simulink model "Red_problema6_Kclasica_v2"  (R2021a)
settings: Solver=ode15s  StartTime=0.0  StopTime=sim_time  RelTol=1e-3
values from neighbouring files (symbols this model uses):
  aE112 = 177.25533427288616    (= 177.255334273)    [data_run_lazo_abierto_simulink.m]    (also in inicializar_areas.m = 179.376259805; script_IMC.m = a112_f)
  aE121 = 28.272251308900536    (= 28.2722513089)    [data_run_lazo_abierto_simulink.m]    (also in inicializar_areas.m; script_IMC.m = a121_f)
  aE213 = 304.960661680865    (= 304.960661681)    [data_run_lazo_abierto_simulink.m]    (also in inicializar_areas.m; script_IMC.m = a213_f)
  aE222 = 104.78323167686085    (= 104.783231677)    [data_run_lazo_abierto_simulink.m]    (also in inicializar_areas.m = 114.075570199; script_IMC.m = a222_f)
  aEcu1 = 2.44278466343862    (= 2.44278466344)    [data_run_lazo_abierto_simulink.m]    (also in inicializar_areas.m = 4.955447053)
  aEcu2 = 9.34130944614368    (= 9.34130944614)    [data_run_lazo_abierto_simulink.m]    (also in inicializar_areas.m = 18.78773145)
  aEhu2 = 53.1053199018638    (= 53.1053199019)    [data_run_lazo_abierto_simulink.m]    (also in inicializar_areas.m = 53.1053199)
  d1_end = 0    [data_run_lazo_abierto_simulink.m]    (also in inicializar_entradas.m; pert_max.m = 0.99; script_build_tfs.m)
  d1_in = 0    [data_run_lazo_abierto_simulink.m]    (also in inicializar_entradas.m; script_build_tfs.m)
  d2_end = 0    [data_run_lazo_abierto_simulink.m]    (also in inicializar_entradas.m; pert_max.m = 0.15; script_build_tfs.m)
  d2_in = 0    [data_run_lazo_abierto_simulink.m]    (also in inicializar_entradas.m; script_build_tfs.m)
  d3_end = 0    [data_run_lazo_abierto_simulink.m]    (also in inicializar_entradas.m; pert_max.m = 0.99; script_build_tfs.m)
  d3_in = 0    [data_run_lazo_abierto_simulink.m]    (also in inicializar_entradas.m; script_build_tfs.m)
  d4_end = 0    [data_run_lazo_abierto_simulink.m]    (also in inicializar_entradas.m; pert_max.m = 0.15; script_build_tfs.m)
  d4_in = 0    [data_run_lazo_abierto_simulink.m]    (also in inicializar_entradas.m; script_build_tfs.m)
  d5_end = 0    [data_run_lazo_abierto_simulink.m]    (also in inicializar_entradas.m; pert_max.m = -0.99; script_build_tfs.m)
  d5_in = 0    [data_run_lazo_abierto_simulink.m]    (also in inicializar_entradas.m; script_build_tfs.m)
  d6_end = 0    [data_run_lazo_abierto_simulink.m]    (also in inicializar_entradas.m; pert_max.m = 0.15; script_build_tfs.m)
  d6_in = 0    [data_run_lazo_abierto_simulink.m]    (also in inicializar_entradas.m; script_build_tfs.m)
  d7_end = 0    [data_run_lazo_abierto_simulink.m]    (also in inicializar_entradas.m; pert_max.m = -0.99; script_build_tfs.m)
  d7_in = 0    [data_run_lazo_abierto_simulink.m]    (also in inicializar_entradas.m; script_build_tfs.m)
  d8_end = 0    [data_run_lazo_abierto_simulink.m]    (also in inicializar_entradas.m; pert_max.m = 0.15; script_build_tfs.m)
  d8_in = 0    [data_run_lazo_abierto_simulink.m]    (also in inicializar_entradas.m; script_build_tfs.m)
  est = 1    [data_run_lazo_abierto_simulink.m]    (also in ini_comun.m; script_build_tfs.m)
  fc1 = 20    [data_run_lazo_abierto_simulink.m]    (also in ini_comun.m; script_build_tfs.m)
  fc2 = 50    [data_run_lazo_abierto_simulink.m]    (also in ini_comun.m; script_build_tfs.m)
  fcu1 = 36    [data_run_lazo_abierto_simulink.m]    (also in ini_comun.m = 1.45; inicializar_areas.m = 1.45; script_build_tfs.m = 1.45)
  fcu2 = 44    [data_run_lazo_abierto_simulink.m]    (also in ini_comun.m = 5; inicializar_areas.m = 5; script_build_tfs.m = 5)
  fh1 = 18    [data_run_lazo_abierto_simulink.m]    (also in ini_comun.m; script_build_tfs.m)
  fh2 = 22    [data_run_lazo_abierto_simulink.m]    (also in ini_comun.m; script_build_tfs.m)
  fhu2 = 14.8    [data_run_lazo_abierto_simulink.m]    (also in ini_comun.m = 15; inicializar_areas.m = 15; script_build_tfs.m = 15)
  hc1 = 1    [data_run_lazo_abierto_simulink.m]    (also in ini_comun.m; script_build_tfs.m)
  hc2 = 1    [data_run_lazo_abierto_simulink.m]    (also in ini_comun.m; script_build_tfs.m)
  hcu = 1    [data_run_lazo_abierto_simulink.m]    (also in ini_comun.m; script_build_tfs.m)
  hh1 = 1    [data_run_lazo_abierto_simulink.m]    (also in ini_comun.m; script_build_tfs.m)
  hh2 = 1    [data_run_lazo_abierto_simulink.m]    (also in ini_comun.m; script_build_tfs.m)
  hhu = 1    [data_run_lazo_abierto_simulink.m]    (also in ini_comun.m; script_build_tfs.m)
  initials = nominales_u_full    [cambiar_estructura.m]    (also in data_run_lazo_abierto_simulink.m; script_build_tfs.m)
  s1 = 30    [data_run_lazo_abierto_simulink.m]    (also in ini_comun.m; script_build_tfs.m)
  switch_var = 2    [script_IMC.m]
  t_step = 2000    [data_run_lazo_abierto_simulink.m]    (also in ini_comun.m = 20000; script_build_tfs.m = 1000)
  Tcin1 = 323    [data_run_lazo_abierto_simulink.m]    (also in ini_comun.m; script_build_tfs.m)
  Tcin2 = 433    [data_run_lazo_abierto_simulink.m]    (also in ini_comun.m; script_build_tfs.m)
  Tcuin = 288    [data_run_lazo_abierto_simulink.m]    (also in ini_comun.m; script_build_tfs.m)
  Thin1 = 543    [data_run_lazo_abierto_simulink.m]    (also in ini_comun.m; script_build_tfs.m)
  Thin2 = 493    [data_run_lazo_abierto_simulink.m]    (also in ini_comun.m; script_build_tfs.m)
  Thuin = 523    [data_run_lazo_abierto_simulink.m]    (also in ini_comun.m; script_build_tfs.m)
libraries: cstblocks x2, simulink x1
(part 1 of 2)
settings Model: Creator=Lautaro  LastModifiedBy=fzpat
settings SolverCC: AlgebraicLoopSolver=TrustRegion
settings DataIOCC: InitialState=xFinal  LimitDataPoints=on  SaveFinalState=on  SaveFormat=Array  ReturnWorkspaceOutputs=off
settings OptimizationCC: BlockReduction=off  BooleanDataType=off  LifeSpan=inf
settings DebuggingCC: SaveWithParameterizedLinksMsg=none  UnderspecifiedInitializationDetection=Classic  MergeDetectMultiDrivingBlocksExec=none  SignalResolutionControl=TryResolveAllWithWarning  SFUnexpectedBacktrackingDiag=warning  SFNoUnconditionalDefaultTransitionDiag=warning  SFExecutionAtInitializationDiag=none  SFMachineParentedDataDiag=warning  ArithmeticOperatorsInVariantConditions=warning
settings HardwareCC: ProdBitPerPointer=32  ProdBitPerSizeT=32  ProdBitPerPtrDiffT=32  ProdLargestAtomicFloat=None  ProdIntDivRoundTo=Undefined  ProdEndianess=Unspecified  ProdWordSize=32  ProdHWDeviceType=32-bit Generic  TargetUnknown=on
settings ModelReferenceCC: PropagateSignalLabelsOutOfModel=off
settings SFSimCC: SimUseLocalCustomCode=off  CustomCodeUndefinedFunction=UseInterfaceOnly
settings RTWCC: RTWUseLocalCustomCode=off
settings CodeAppCC: StateflowObjectComments=on
settings GRTTargetCC: TargetLangStandard=C89/C90 (ANSI)
settings ConfigComp: CovMetricSettings=dw  CovSaveCumulativeToWorkspaceVar=on  CovSaveSingleToWorkspaceVar=on  CovExternalEMLEnable=off  CovSFcnEnable=off

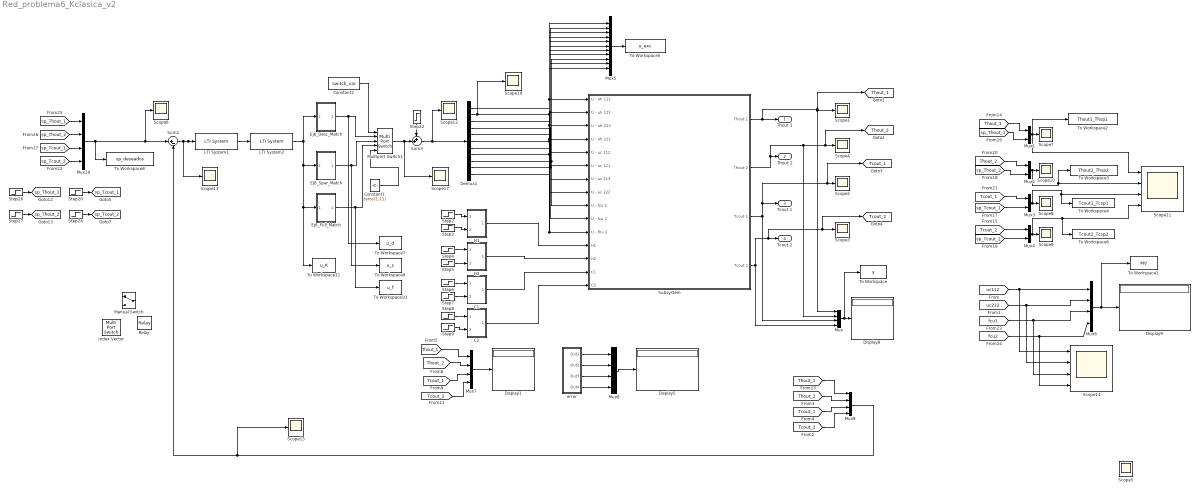
== system Red_problema6_Kclasica_v2 ==
  C1 : Subsystem
  "C2 " : Subsystem
  Constant1 : Constant  Value=zeros(1,11)
  Constant2 : Constant  Value=switch_var
  Demux1 : Demux  Outputs=11
  Display{1,5,8..9} (4 alike) : Display
  Ej6_Desc_Match : Subsystem
  Ej6_Full_Match : Subsystem
  Ej6_Spar_Match : Subsystem
  "H1 " : Subsystem
  H2 : Subsystem
  Index Vector : MultiPortSwitch  DataPortOrder=Zero-based contiguous  Inputs=1  zeroidx=on
  LTI System1 : cstblocks/LTI System  sys=Kimc_u  IC=[]
  LTI System2 : cstblocks/LTI System  sys=K_clasica_2  IC=[]
  Manual Switch : ManualSwitch
  Multiport Switch1 : MultiPortSwitch  DataPortOrder=Zero-based contiguous  DataPortForDefault=Additional data port  DiagnosticForDefault=None  zeroidx=on
  Mux{,6..10} (6 alike) : Mux
  Mux{1..4} (4 alike) : Mux  Inputs=2
  Mux5 : Mux  Inputs=11
  Relay : Relay
  Scope{1..10,12..13,15,17,19} (15 alike) : Scope
  Scope11 : Scope  NumInputPorts=4
  Scope14 : Scope  NumInputPorts=4
  Step2 : Step  Time=t_step  Before=d1_in  After=d1_end
  Step20 : Step  Time=1e9  Before=210+273  After=210+273
  Step22 : Step  Time=0  Before=initials  After=initials
  Step24 : Step  Time=1e10  Before=210+273  After=210+273
  Step26 : Step  Time=1e9  Before=160+273  After=160+273
  Step27 : Step  Time=1e9  Before=60+273  After=60+273
  Step3 : Step  Time=t_step  Before=d2_in  After=d2_end
  Step4 : Step  Time=t_step  Before=d3_in  After=d3_end
  Step5 : Step  Time=t_step  Before=d4_in  After=d4_end
  Step6 : Step  Time=t_step  Before=d5_in  After=d5_end
  Step7 : Step  Time=t_step  Before=d6_in  After=d6_end
  Step8 : Step  Time=t_step  Before=d7_in  After=d7_end
  Step9 : Step  Time=t_step  Before=d8_in  After=d8_end
  Subsystem : Subsystem
  Sum1 : Sum  Inputs=|+-
  Sum3 : Sum  Inputs=++|
  To Workspace : ToWorkspace  VariableName=y  SaveFormat=Timeseries  SampleTime=-1
  To Workspace1 : ToWorkspace  VariableName=MV  SaveFormat=Timeseries  SampleTime=-1
  To Workspace10 : ToWorkspace  VariableName=u_f  SaveFormat=Timeseries  SampleTime=-1
      settings: Save2DSignal=2-D array (concatenate along first dimension)
  To Workspace11 : ToWorkspace  VariableName=u_K  SaveFormat=Timeseries  SampleTime=-1
      settings: Save2DSignal=2-D array (concatenate along first dimension)
  To Workspace2 : ToWorkspace  VariableName=Thout1_Thsp1  SaveFormat=Timeseries  SampleTime=-1
  To Workspace3 : ToWorkspace  VariableName=Thout2_Thsp2  SampleTime=-1
  To Workspace4 : ToWorkspace  VariableName=Tcout1_Tcsp1  SampleTime=-1
  To Workspace5 : ToWorkspace  VariableName=u_exc  SaveFormat=Timeseries  SampleTime=-1
      settings: Save2DSignal=2-D array (concatenate along first dimension)
  To Workspace6 : ToWorkspace  VariableName=Tcout2_Tcsp2  SampleTime=-1
  To Workspace7 : ToWorkspace  VariableName=u_d  SaveFormat=Timeseries  SampleTime=-1
      settings: Save2DSignal=2-D array (concatenate along first dimension)
  To Workspace8 : ToWorkspace  VariableName=sp_deseados  SampleTime=-1
  To Workspace9 : ToWorkspace  VariableName=u_s  SaveFormat=Timeseries  SampleTime=-1
      settings: Save2DSignal=2-D array (concatenate along first dimension)
  error : Subsystem
  Thout 1 : Outport  VectorParamsAs1DForOutWhenUnconnected=off
  Thout 2 : Outport  Port=2  VectorParamsAs1DForOutWhenUnconnected=off
  Tcout 1 : Outport  Port=3  VectorParamsAs1DForOutWhenUnconnected=off
  Tcout 2 : Outport  Port=4  VectorParamsAs1DForOutWhenUnconnected=off
  tag scope: Tcout_1=global, Tcout_2=global, Thout_1=global, Thout_2=global, sp_Tcout_1=global, sp_Tcout_2=global, sp_Thout_1=global, sp_Thout_2=global
  wires:
  Subsystem/1(Thout 1) -> Mux/1, Scope1/1, [Thout_1], Thout 1/1
  Mux/1 -> To Workspace/1, Display8/1
  "H1 "/1(Out1) -> Subsystem/12(H1)
  H2/1(Out1) -> Subsystem/13(H2)
  C1/1(Out1) -> Subsystem/14(C1)
  "C2 "/1(Out1) -> Subsystem/15(C2)
  Subsystem/2(Thout 2) -> [Thout_2], Scope4/1, Mux/2, Thout 2/1
  Subsystem/3(Tcout 1) -> [Tcout_1], Scope2/1, Tcout 1/1, Mux/3
  Step2/1 -> "H1 "/1(Thin 1)
  Step3/1 -> "H1 "/2(fhin 1)
  Step4/1 -> H2/1(Thin 2)
  Step5/1 -> H2/2(fhin 2)
  Step6/1 -> C1/1(Tcin 1)
  Step7/1 -> C1/2(fcin 1)
  Step8/1 -> "C2 "/1(Tcin 2)
  Step9/1 -> "C2 "/2(fcin 2)
  Demux1/1 -> Mux5/1, Subsystem/1(U - uh 112)
  Demux1/11 -> Mux5/11, Subsystem/11(U - fhu 2)
  Demux1/2 -> Scope19/1, Mux5/5, Subsystem/5(U - uc 112)
  Demux1/9 -> Mux5/9, Subsystem/9(U - fcu 1)
  Subsystem/4(Tcout 2) -> [Tcout_2], Scope3/1, Tcout 2/1, Mux/4
  Demux1/10 -> Mux5/10, Subsystem/10(U - fcu 2)
  Demux1/6 -> Subsystem/7(U - uc 213), Mux5/7
  Demux1/5 -> Mux5/3, Subsystem/3(U - uh 213)
  Mux7/1 -> Display1/1
  [Thout_1] -> Mux7/1
  [Thout_2] -> Mux7/2
  [Tcout_1] -> Mux7/3
  [Tcout_2] -> Mux7/4
  Mux8/1 -> Display5/1
  error/1(Out1) -> Mux8/1
  error/2(Out2) -> Mux8/2
  error/3(Out3) -> Mux8/3
  error/4(Out4) -> Mux8/4
  Mux6/1 -> To Workspace1/1, Display9/1
  [uc112] -> Mux6/1, Scope14/1
  [uc222] -> Mux6/2, Scope14/2
  [fcu1] -> Mux6/3, Scope14/3
  [fcu2] -> Scope14/4, Mux6/4
  Mux1/1 -> To Workspace2/1, Scope11/1, Scope7/1
  [sp_Thout_1] -> Mux1/2
  Mux2/1 -> To Workspace3/1, Scope11/2, Scope10/1
  [sp_Thout_2] -> Mux2/2
  Mux3/1 -> To Workspace4/1, Scope11/3, Scope8/1
  [sp_Tcout_1] -> Mux3/2
  Mux4/1 -> To Workspace6/1, Scope11/4, Scope9/1
  [sp_Tcout_2] -> Mux4/2
  [Thout_1] -> Mux1/1
  [Thout_2] -> Mux2/1
  [Tcout_1] -> Mux3/1
  [Tcout_2] -> Mux4/1
  Step20/1 -> [sp_Tcout_1]
  Step24/1 -> [sp_Tcout_2]
  Step26/1 -> [sp_Thout_1]
  Step27/1 -> [sp_Thout_2]
  Demux1/3 -> Mux5/2, Subsystem/2(U - uh 121)
  Demux1/7 -> Mux5/4, Subsystem/4(U - uh 222)
  Demux1/4 -> Mux5/6, Subsystem/6(U - uc 121)
  Demux1/8 -> Mux5/8, Subsystem/8(U - uc 222)
  Mux5/1 -> To Workspace5/1
  [Thout_1] -> Mux9/1
  [Thout_2] -> Mux9/2
  [Tcout_2] -> Mux9/4
  [Tcout_1] -> Mux9/3
  Sum1/1 -> Scope13/1, LTI System1/1
  Mux9/1 -> Sum1/2, Scope15/1
  Mux10/1 -> Scope6/1, Sum1/1, To Workspace8/1
  [sp_Thout_1] -> Mux10/1
  [sp_Thout_2] -> Mux10/2
  [sp_Tcout_1] -> Mux10/3
  [sp_Tcout_2] -> Mux10/4
  Constant2/1 -> Multiport Switch1/1
  LTI System1/1 -> LTI System2/1
  Ej6_Desc_Match/1(Out1) -> To Workspace7/1, Multiport Switch1/2
  Ej6_Spar_Match/1(Out1) -> To Workspace9/1, Multiport Switch1/3
  Sum3/1 -> Demux1/1, Scope12/1
  Step22/1 -> Sum3/1
  Multiport Switch1/1 -> Scope17/1, Sum3/2
  Ej6_Full_Match/1(Out1) -> To Workspace10/1, Multiport Switch1/4
  Constant1/1 -> Multiport Switch1/5
  LTI System2/1 -> To Workspace11/1, Ej6_Full_Match/1(In1), Ej6_Spar_Match/1(In1), Ej6_Desc_Match/1(In1)

== system Red_problema6_Kclasica_v2/C1 ==
  Tcin 1 : Inport
  fcin 1 : Inport  Port=2
  Add2 : Sum
  Add3 : Sum
  Constant3 : Constant  Value=Tcin1
  Constant4 : Constant  Value=fc1
  Mux5 : Mux  Inputs=3
  hc : Step  Before=hc1  After=hc1
  valvula : Subsystem
  Out1 : Outport  VectorParamsAs1DForOutWhenUnconnected=off
  wires:
  Constant3/1 -> Add2/1
  Constant4/1 -> Add3/1
  Tcin 1/1 -> Add2/2
  fcin 1/1 -> Add3/2
  Add2/1 -> Mux5/1
  Add3/1 -> Mux5/2
  hc/1 -> Mux5/3
  Mux5/1 -> valvula/1(In1)
  valvula/1(Out1) -> Out1/1

== system Red_problema6_Kclasica_v2/C2  ==
  Tcin 2 : Inport
  fcin 2 : Inport  Port=2
  Add4 : Sum
  Add5 : Sum
  Constant5 : Constant  Value=Tcin2
  Constant6 : Constant  Value=fc2
  Mux5 : Mux  Inputs=3
  hc : Step  Before=hc2  After=hc2
  valvula : Subsystem
  Out1 : Outport  VectorParamsAs1DForOutWhenUnconnected=off
  wires:
  Constant5/1 -> Add4/1
  Constant6/1 -> Add5/1
  Tcin 2/1 -> Add4/2
  fcin 2/1 -> Add5/2
  Add4/1 -> Mux5/1
  Add5/1 -> Mux5/2
  hc/1 -> Mux5/3
  Mux5/1 -> valvula/1(In1)
  valvula/1(Out1) -> Out1/1

== system Red_problema6_Kclasica_v2/Ej6_Desc_Match ==
  In1 : Inport
  Constant1 : Constant  Value=0
  Constant2 : Constant  Value=0
  Demux3 : Demux
  Gain : Gain
  Mux10 : Mux  Inputs=11
  Out1 : Outport
  wires:
  In1/1 -> Demux3/1
  Constant2/1 -> Mux10/8, Mux10/7, Mux10/6, Mux10/3, Mux10/4, Mux10/5
  Constant1/1 -> Mux10/1
  Demux3/4 -> Mux10/11
  Demux3/3 -> Gain/1
  Demux3/2 -> Mux10/10
  Demux3/1 -> Mux10/9
  Mux10/1 -> Out1/1
  Gain/1 -> Mux10/2

== system Red_problema6_Kclasica_v2/Ej6_Full_Match ==
  In1 : Inport
  Constant1 : Constant  Value=0
  Constant2 : Constant  Value=0
  Constant3 : Constant  Value=0
  Demux3 : Demux
  Mux10 : Mux  Inputs=11
  Out1 : Outport
  wires:
  Constant3/1 -> Mux10/11
  In1/1 -> Demux3/1
  Constant2/1 -> Mux10/7, Mux10/4, Mux10/3, Mux10/5, Mux10/6
  Constant1/1 -> Mux10/1
  Demux3/4 -> Mux10/8
  Demux3/3 -> Mux10/2
  Demux3/2 -> Mux10/10
  Demux3/1 -> Mux10/9
  Mux10/1 -> Out1/1

== system Red_problema6_Kclasica_v2/Ej6_Spar_Match ==
  In1 : Inport
  Constant1 : Constant  Value=0
  Constant2 : Constant  Value=0
  Constant3 : Constant  Value=0
  Demux3 : Demux
  Mux10 : Mux  Inputs=11
  Out1 : Outport
  wires:
  Mux10/1 -> Out1/1
  Demux3/1 -> Mux10/9
  Demux3/2 -> Mux10/10
  Demux3/3 -> Mux10/3
  Demux3/4 -> Mux10/8
  Constant1/1 -> Mux10/2, Mux10/1
  Constant2/1 -> Mux10/6, Mux10/5, Mux10/4, Mux10/7
  In1/1 -> Demux3/1
  Constant3/1 -> Mux10/11

== system Red_problema6_Kclasica_v2/H1  ==
  Thin 1 : Inport
  fhin 1 : Inport  Port=2
  Add : Sum
  Add1 : Sum
  Constant1 : Constant  Value=Thin1
  Constant2 : Constant  Value=fh1
  Mux5 : Mux  Inputs=3
  hh : Step  Before=hh1  After=hh1
  valvula : Subsystem
  Out1 : Outport  VectorParamsAs1DForOutWhenUnconnected=off
  wires:
  Constant1/1 -> Add/1
  Thin 1/1 -> Add/2
  Add/1 -> Mux5/1
  Constant2/1 -> Add1/1
  fhin 1/1 -> Add1/2
  hh/1 -> Mux5/3
  Add1/1 -> Mux5/2
  Mux5/1 -> valvula/1(In1)
  valvula/1(Out1) -> Out1/1

== system Red_problema6_Kclasica_v2/H2 ==
  Thin 2 : Inport
  fhin 2 : Inport  Port=2
  Add : Sum
  Add1 : Sum
  Constant1 : Constant  Value=Thin2
  Constant2 : Constant  Value=fh2
  Mux5 : Mux  Inputs=3
  hh : Step  Before=hh2  After=hh2
  valvula : Subsystem
  Out1 : Outport  VectorParamsAs1DForOutWhenUnconnected=off
  wires:
  Constant1/1 -> Add/1
  Thin 2/1 -> Add/2
  Add/1 -> Mux5/1
  Constant2/1 -> Add1/1
  fhin 2/1 -> Add1/2
  hh/1 -> Mux5/3
  Add1/1 -> Mux5/2
  Mux5/1 -> valvula/1(In1)
  valvula/1(Out1) -> Out1/1

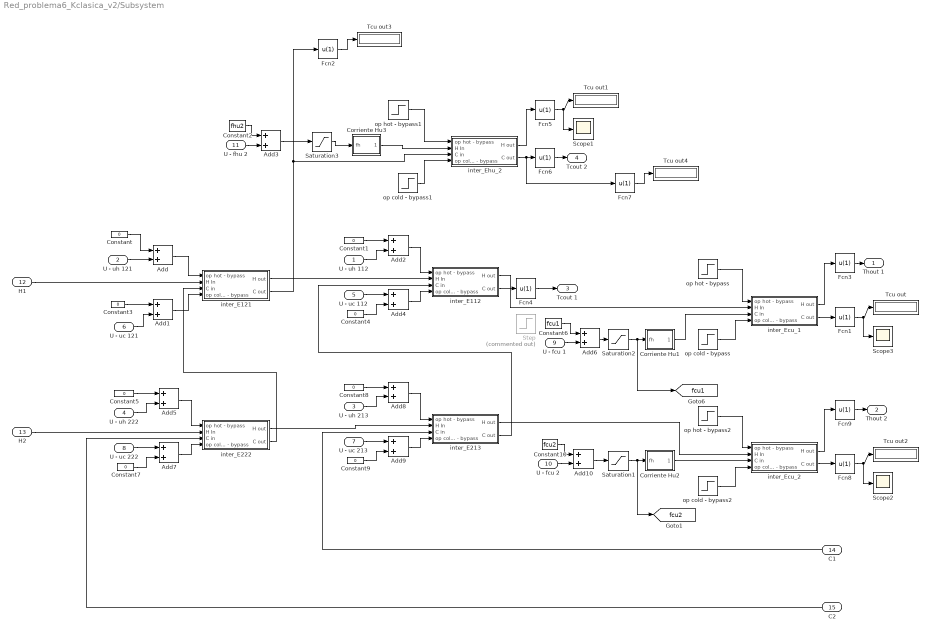
== system Red_problema6_Kclasica_v2/Subsystem ==
  U - uh 112 : Inport
  U - uh 121 : Inport  Port=2
  U - uh 213 : Inport  Port=3
  U - uh 222 : Inport  Port=4
  U - uc 112 : Inport  Port=5
  U - uc 121 : Inport  Port=6
  U - uc 213 : Inport  Port=7
  U - uc 222 : Inport  Port=8
  U - fcu 1 : Inport  Port=9
  U - fcu 2 : Inport  Port=10
  U - fhu 2 : Inport  Port=11
  H1 : Inport  Port=12
  H2 : Inport  Port=13
  C1 : Inport  Port=14
  C2 : Inport  Port=15
  Add{,1..10} (11 alike) : Sum
  Constant{,1,3..5,7..9} (8 alike) : Constant  Value=0
  Constant10 : Constant  Value=fcu2
  Constant2 : Constant  Value=fhu2
  Constant6 : Constant  Value=fcu1
  Corriente Hu1 : Subsystem
  Corriente Hu2 : Subsystem
  Corriente Hu3 : Subsystem
  Fcn{1..9} (9 alike) : Fcn  Expr=u(1)
  Saturation1 : Saturate  UpperLimit=1e9  LowerLimit=0
  Saturation2 : Saturate  UpperLimit=1e9  LowerLimit=0
  Saturation3 : Saturate  UpperLimit=1e9  LowerLimit=0
  Scope1 : Scope
  Scope2 : Scope
  Scope3 : Scope
  Step : Step  Commented=on  Time=2000  Before=fcu1  After=fcu1+30  SampleTime=0
  Tcu out{,1..4} (5 alike) : Display
  inter_E112 : Subsystem
  inter_E121 : Subsystem
  inter_E213 : Subsystem
  inter_E222 : Subsystem
  inter_Ecu_1 : Subsystem
  inter_Ecu_2 : Subsystem
  inter_Ehu_2 : Subsystem
  op cold - bypass : Step  Time=0  After=0  SampleTime=0
  op cold - bypass1 : Step  Time=0  After=0  SampleTime=0
  op cold - bypass2 : Step  Time=0  After=0  SampleTime=0
  op hot - bypass : Step  Time=0  After=0  SampleTime=0
  op hot - bypass1 : Step  Time=0  After=0  SampleTime=0
  op hot - bypass2 : Step  Time=0  After=0  SampleTime=0
  Thout 1 : Outport  VectorParamsAs1DForOutWhenUnconnected=off
  Thout 2 : Outport  Port=2  VectorParamsAs1DForOutWhenUnconnected=off
  Tcout 1 : Outport  Port=3  VectorParamsAs1DForOutWhenUnconnected=off
  Tcout 2 : Outport  Port=4  VectorParamsAs1DForOutWhenUnconnected=off
  tag scope: fcu1=global, fcu2=global
  wires:
  op cold - bypass/1 -> inter_Ecu_1/4("op cold - bypass ")
  Fcn1/1 -> Scope3/1, Tcu out/1
  op hot - bypass/1 -> inter_Ecu_1/1("op hot - bypass ")
  U - uh 121/1 -> Add/2
  Constant/1 -> Add/1
  U - uc 121/1 -> Add1/2
  Add1/1 -> inter_E121/4("op cold - bypass ")
  Add/1 -> inter_E121/1("op hot - bypass ")
  U - uh 112/1 -> Add2/2
  Constant1/1 -> Add2/1
  Add2/1 -> inter_E112/1("op hot - bypass ")
  Constant3/1 -> Add1/1
  U - uc 112/1 -> Add4/1
  Constant4/1 -> Add4/2
  Add4/1 -> inter_E112/4("op cold - bypass ")
  Add6/1 -> Saturation2/1
  U - fcu 1/1 -> Add6/2
  op cold - bypass1/1 -> inter_Ehu_2/4("op cold - bypass ")
  Fcn5/1 -> Scope1/1, Tcu out1/1
  op hot - bypass1/1 -> inter_Ehu_2/1("op hot - bypass ")
  Add3/1 -> Saturation3/1
  U - fhu 2/1 -> Add3/2
  Constant2/1 -> Add3/1
  Corriente Hu3/1(Out1) -> inter_Ehu_2/2(H In)
  inter_Ehu_2/1(H out) -> Fcn5/1
  Fcn4/1 -> Tcout 1/1
  Fcn6/1 -> Tcout 2/1
  Fcn3/1 -> Thout 1/1
  inter_E121/1(H out) -> inter_E112/2(H In)
  Corriente Hu1/1(Out1) -> inter_Ecu_1/3(C in)
  inter_Ecu_1/2(C out) -> Fcn1/1
  inter_Ecu_1/1(H out) -> Fcn3/1
  U - uh 222/1 -> Add5/2
  Constant5/1 -> Add5/1
  Add5/1 -> inter_E222/1("op hot - bypass ")
  U - uc 222/1 -> Add7/1
  Constant7/1 -> Add7/2
  Add7/1 -> inter_E222/4("op cold - bypass ")
  U - uh 213/1 -> Add8/2
  Constant8/1 -> Add8/1
  Add8/1 -> inter_E213/1("op hot - bypass ")
  U - uc 213/1 -> Add9/1
  Constant9/1 -> Add9/2
  Add9/1 -> inter_E213/4("op cold - bypass ")
  H2/1 -> inter_E222/2(H In)
  inter_E222/1(H out) -> inter_E213/2(H In)
  op cold - bypass2/1 -> inter_Ecu_2/4("op cold - bypass ")
  Fcn8/1 -> Scope2/1, Tcu out2/1
  op hot - bypass2/1 -> inter_Ecu_2/1("op hot - bypass ")
  Add10/1 -> Saturation1/1
  U - fcu 2/1 -> Add10/2
  Constant10/1 -> Add10/1
  Fcn9/1 -> Thout 2/1
  Corriente Hu2/1(Out1) -> inter_Ecu_2/3(C in)
  inter_E213/1(H out) -> inter_Ecu_2/2(H In)
  inter_Ecu_2/2(C out) -> Fcn8/1
  inter_Ecu_2/1(H out) -> Fcn9/1
  C1/1 -> inter_E213/3(C in)
  C2/1 -> inter_E222/3(C in)
  inter_E121/2(C out) -> Fcn2/1, inter_Ehu_2/3(C in)
  Saturation3/1 -> Corriente Hu3/1(fh)
  Saturation2/1 -> [fcu1], Corriente Hu1/1(fh)
  Saturation1/1 -> [fcu2], Corriente Hu2/1(fh)
  Fcn2/1 -> Tcu out3/1
  inter_Ehu_2/2(C out) -> Fcn7/1, Fcn6/1
  Fcn7/1 -> Tcu out4/1
  H1/1 -> inter_E121/2(H In)
  inter_E222/2(C out) -> inter_E121/3(C in)
  inter_E112/1(H out) -> inter_Ecu_1/2(H In)
  inter_E112/2(C out) -> Fcn4/1
  inter_E213/2(C out) -> inter_E112/3(C in)
  Constant6/1 -> Add6/1

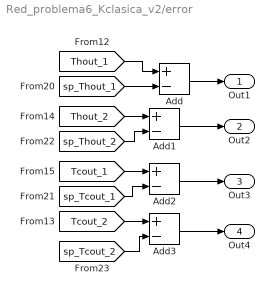
== system Red_problema6_Kclasica_v2/error ==
  Add{,1..3} (4 alike) : Sum  Inputs=+-
  Out1 : Outport  VectorParamsAs1DForOutWhenUnconnected=off
  Out2 : Outport  Port=2  VectorParamsAs1DForOutWhenUnconnected=off
  Out3 : Outport  Port=3  VectorParamsAs1DForOutWhenUnconnected=off
  Out4 : Outport  Port=4  VectorParamsAs1DForOutWhenUnconnected=off
  wires:
  [sp_Thout_2] -> Add1/2
  [sp_Tcout_2] -> Add3/2
  [sp_Tcout_1] -> Add2/2
  [sp_Thout_1] -> Add/2
  [Thout_2] -> Add1/1
  [Thout_1] -> Add/1
  [Tcout_1] -> Add2/1
  [Tcout_2] -> Add3/1
  Add1/1 -> Out2/1
  Add/1 -> Out1/1
  Add3/1 -> Out4/1
  Add2/1 -> Out3/1

== system Red_problema6_Kclasica_v2/C1/valvula ==
  In1 : Inport
  Gain : Gain  Gain=s1
  Gain1 : Gain  Gain=s1
  Integrator : Integrator  InitialCondition=[Tcin1 fc1 hc1]
  Sum : Sum  Inputs=|+-
  Out1 : Outport  VectorParamsAs1DForOutWhenUnconnected=off
  wires:
  Gain1/1 -> Sum/2
  Integrator/1 -> Gain1/1, Out1/1
  Sum/1 -> Integrator/1
  Gain/1 -> Sum/1
  In1/1 -> Gain/1

== system Red_problema6_Kclasica_v2/C2 /valvula ==
  In1 : Inport
  Gain : Gain  Gain=s1
  Gain1 : Gain  Gain=s1
  Integrator : Integrator  InitialCondition=[Tcin2 fc2 hc2]
  Sum : Sum  Inputs=|+-
  Out1 : Outport  VectorParamsAs1DForOutWhenUnconnected=off
  wires:
  Gain1/1 -> Sum/2
  Integrator/1 -> Out1/1, Gain1/1
  Sum/1 -> Integrator/1
  Gain/1 -> Sum/1
  In1/1 -> Gain/1

== system Red_problema6_Kclasica_v2/H1 /valvula ==
  In1 : Inport
  Gain : Gain  Gain=s1
  Gain1 : Gain  Gain=s1
  Integrator : Integrator  InitialCondition=[Thin1 fh1 hh1]
  Sum : Sum  Inputs=|+-
  Out1 : Outport  VectorParamsAs1DForOutWhenUnconnected=off
  wires:
  Gain1/1 -> Sum/2
  Integrator/1 -> Gain1/1, Out1/1
  Sum/1 -> Integrator/1
  Gain/1 -> Sum/1
  In1/1 -> Gain/1

== system Red_problema6_Kclasica_v2/H2/valvula ==
  In1 : Inport
  Gain : Gain  Gain=s1
  Gain1 : Gain  Gain=s1
  Integrator : Integrator  InitialCondition=[Thin2 fh2 hh2]
  Sum : Sum  Inputs=|+-
  Out1 : Outport  VectorParamsAs1DForOutWhenUnconnected=off
  wires:
  Gain1/1 -> Sum/2
  Integrator/1 -> Gain1/1, Out1/1
  Sum/1 -> Integrator/1
  Gain/1 -> Sum/1
  In1/1 -> Gain/1

== system Red_problema6_Kclasica_v2/Subsystem/Corriente Hu1 ==
  fh : Inport
  Mux5 : Mux  Inputs=3
  hh : Step  Before=1  SampleTime=0
  th : Step  Time=2  Before=15+273  After=15+273  SampleTime=0
  valvula 3 : Subsystem
  Out1 : Outport  VectorParamsAs1DForOutWhenUnconnected=off
  wires:
  hh/1 -> Mux5/3
  th/1 -> Mux5/1
  fh/1 -> Mux5/2
  Mux5/1 -> valvula 3/1(In1)
  valvula 3/1(Out1) -> Out1/1

== system Red_problema6_Kclasica_v2/Subsystem/Corriente Hu2 ==
  fh : Inport
  Mux5 : Mux  Inputs=3
  hh : Step  Before=1  SampleTime=0
  th : Step  Time=2  Before=15+273  After=15+273  SampleTime=0
  valvula 3 : Subsystem
  Out1 : Outport  VectorParamsAs1DForOutWhenUnconnected=off
  wires:
  hh/1 -> Mux5/3
  th/1 -> Mux5/1
  fh/1 -> Mux5/2
  Mux5/1 -> valvula 3/1(In1)
  valvula 3/1(Out1) -> Out1/1

== system Red_problema6_Kclasica_v2/Subsystem/Corriente Hu3 ==
  fh : Inport
  Mux5 : Mux  Inputs=3
  hh : Step  Before=1  SampleTime=0
  th : Step  Time=2  Before=250+273  After=250+273  SampleTime=0
  valvula 3 : Subsystem
  Out1 : Outport  VectorParamsAs1DForOutWhenUnconnected=off
  wires:
  hh/1 -> Mux5/3
  th/1 -> Mux5/1
  fh/1 -> Mux5/2
  Mux5/1 -> valvula 3/1(In1)
  valvula 3/1(Out1) -> Out1/1

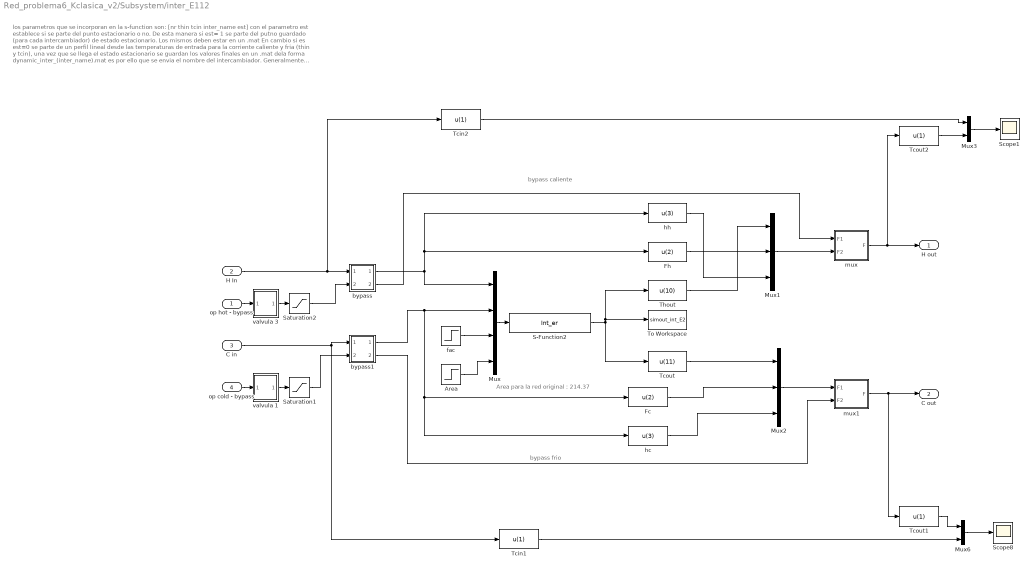
== system Red_problema6_Kclasica_v2/Subsystem/inter_E112 ==
  note: Area para la red original : 214.37
  note: bypass caliente
  note: bypass frio
  note: los parametros que se incorporan en la s-function son: [nr thin tcin inter_name est]
      | con el parametro est establece si se parte del punto estacionario o no. De esta manera si est= 1 se parte del putno guardado (para cada intercambiador) de estado estacionario. Los mismos deben estar en un .mat
      | En cambio si es est=0 se parte de un perfil lineal  desde las temperaturas de entrada para la corriente caliente y fria (thin y tcin), una vez que se llega el estado estacionario se guardan los valores finales en un .mat
      | dela forma dynamic_inter_(inter_name).mat   es por ello que se envia el nombre del intercambiador.
      | Generalmente para la primera vez que se corre la red se una est=0 para que llegue al estado estacionario y una vez que se alcanzó se vuelve a correr con est= 1 para hacer análisis de control
  "op hot - bypass " : Inport
  H In : Inport  Port=2
  C in : Inport  Port=3
  "op cold - bypass " : Inport  Port=4
  Area : Step  Time=8  Before=aE112  After=aE112  SampleTime=0
  Fc : Fcn  Expr=u(2)
  Fh : Fcn  Expr=u(2)
  Mux : Mux
  Mux1 : Mux  Inputs=3
  Mux2 : Mux  Inputs=3
  Mux3 : Mux  Inputs=2
  Mux6 : Mux  Inputs=2
  S-Function2 : S-Function  FunctionName=Int_er  Parameters=10 528.5 433 112 est  SFunctionDeploymentMode=off  EnableBusSupport=off
  Saturation1 : Saturate  UpperLimit=1  LowerLimit=0
  Saturation2 : Saturate  UpperLimit=1  LowerLimit=0
  Scope1 : Scope
  Scope8 : Scope
  Tcin1 : Fcn  Expr=u(1)
  Tcin2 : Fcn  Expr=u(1)
  Tcout : Fcn  Expr=u(11)
  Tcout1 : Fcn  Expr=u(1)
  Tcout2 : Fcn  Expr=u(1)
  Thout : Fcn  Expr=u(10)
  To Workspace : ToWorkspace  VariableName=simout_int_E2  SampleTime=-1
  bypass : Subsystem
  bypass1 : Subsystem
  fac : Step  After=0  SampleTime=0
  hc : Fcn  Expr=u(3)
  hh : Fcn  Expr=u(3)
  mux : Subsystem
  mux1 : Subsystem
  valvula 1 : Subsystem
  valvula 3 : Subsystem
  H out : Outport  VectorParamsAs1DForOutWhenUnconnected=off
  C out : Outport  Port=2  VectorParamsAs1DForOutWhenUnconnected=off
  wires:
  Tcin2/1 -> Mux3/1
  Tcout2/1 -> Mux3/2
  Mux3/1 -> Scope1/1
  Tcin1/1 -> Mux6/2
  Tcout1/1 -> Mux6/1
  Mux6/1 -> Scope8/1
  bypass1/2(" 2") -> mux1/2(F2)
  bypass1/1(" 1") -> Mux/2, Fc/1, hc/1
  mux1/1("F ") -> C out/1, Tcout1/1
  Mux2/1 -> mux1/1(F1)
  mux/1("F ") -> H out/1, Tcout2/1
  C in/1 -> bypass1/1(1), Tcin1/1
  bypass/2(" 2") -> mux/1(F1)
  Mux1/1 -> mux/2(F2)
  bypass/1(" 1") -> hh/1, Fh/1, Mux/1
  H In/1 -> bypass/1(1), Tcin2/1
  Area/1 -> Mux/4
  hh/1 -> Mux1/3
  hc/1 -> Mux2/3
  fac/1 -> Mux/3
  Mux/1 -> S-Function2/1
  S-Function2/1 -> Tcout/1, To Workspace/1, Thout/1
  Fh/1 -> Mux1/2
  Fc/1 -> Mux2/2
  Thout/1 -> Mux1/1
  Tcout/1 -> Mux2/1
  Saturation1/1 -> bypass1/2(u122)
  Saturation2/1 -> bypass/2(u122)
  "op hot - bypass "/1 -> valvula 3/1(In1)
  "op cold - bypass "/1 -> valvula 1/1(In1)
  valvula 3/1(Out1) -> Saturation2/1
  valvula 1/1(Out1) -> Saturation1/1

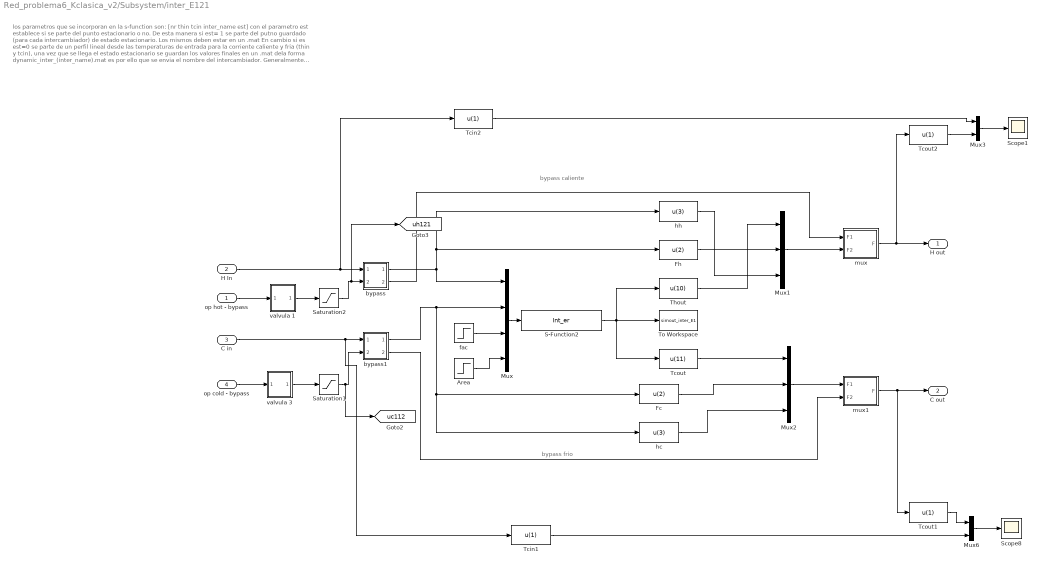
== system Red_problema6_Kclasica_v2/Subsystem/inter_E121 ==
  note: los parametros que se incorporan en la s-function son: [nr thin tcin inter_name est]
      | con el parametro est establece si se parte del punto estacionario o no. De esta manera si est= 1 se parte del putno guardado (para cada intercambiador) de estado estacionario. Los mismos deben estar en un .mat
      | En cambio si es est=0 se parte de un perfil lineal  desde las temperaturas de entrada para la corriente caliente y fria (thin y tcin), una vez que se llega el estado estacionario se guardan los valores finales en un .mat
      | dela forma dynamic_inter_(inter_name).mat   es por ello que se envia el nombre del intercambiador.
      | Generalmente para la primera vez que se corre la red se una est=0 para que llegue al estado estacionario y una vez que se alcanzó se vuelve a correr con est= 1 para hacer análisis de control
  note: bypass frio
  note: bypass caliente
  "op hot - bypass " : Inport
  H In : Inport  Port=2
  C in : Inport  Port=3
  "op cold - bypass " : Inport  Port=4
  Area : Step  Time=0  Before=aE121  After=aE121  SampleTime=0
  Fc : Fcn  Expr=u(2)
  Fh : Fcn  Expr=u(2)
  Mux : Mux
  Mux1 : Mux  Inputs=3
  Mux2 : Mux  Inputs=3
  Mux3 : Mux  Inputs=2
  Mux6 : Mux  Inputs=2
  S-Function2 : S-Function  FunctionName=Int_er  Parameters=10 543 455 121 est  SFunctionDeploymentMode=off  EnableBusSupport=off
  Saturation1 : Saturate  UpperLimit=1  LowerLimit=0
  Saturation2 : Saturate  UpperLimit=1  LowerLimit=0
  Scope1 : Scope
  Scope8 : Scope
  Tcin1 : Fcn  Expr=u(1)
  Tcin2 : Fcn  Expr=u(1)
  Tcout : Fcn  Expr=u(11)
  Tcout1 : Fcn  Expr=u(1)
  Tcout2 : Fcn  Expr=u(1)
  Thout : Fcn  Expr=u(10)
  To Workspace : ToWorkspace  VariableName=simout_inter_E1  SampleTime=-1
  bypass : Subsystem
  bypass1 : Subsystem
  fac : Step  After=0  SampleTime=0
  hc : Fcn  Expr=u(3)
  hh : Fcn  Expr=u(3)
  mux : Subsystem
  mux1 : Subsystem
  valvula 1 : Subsystem
  valvula 3 : Subsystem
  H out : Outport  VectorParamsAs1DForOutWhenUnconnected=off
  C out : Outport  Port=2  VectorParamsAs1DForOutWhenUnconnected=off
  tag scope: uc112=global, uh121=global
  wires:
  Tcout/1 -> Mux2/1
  Thout/1 -> Mux1/1
  Fc/1 -> Mux2/2
  Fh/1 -> Mux1/2
  S-Function2/1 -> Thout/1, To Workspace/1, Tcout/1
  Mux/1 -> S-Function2/1
  fac/1 -> Mux/3
  hc/1 -> Mux2/3
  hh/1 -> Mux1/3
  Area/1 -> Mux/4
  H In/1 -> Tcin2/1, bypass/1(1)
  bypass/1(" 1") -> Mux/1, Fh/1, hh/1
  Mux1/1 -> mux/2(F2)
  bypass/2(" 2") -> mux/1(F1)
  C in/1 -> Tcin1/1, bypass1/1(1)
  mux/1("F ") -> Tcout2/1, H out/1
  Mux2/1 -> mux1/1(F1)
  mux1/1("F ") -> Tcout1/1, C out/1
  bypass1/1(" 1") -> hc/1, Fc/1, Mux/2
  bypass1/2(" 2") -> mux1/2(F2)
  Mux6/1 -> Scope8/1
  Tcout1/1 -> Mux6/1
  Tcin1/1 -> Mux6/2
  Mux3/1 -> Scope1/1
  Tcout2/1 -> Mux3/2
  Tcin2/1 -> Mux3/1
  Saturation1/1 -> [uc112], bypass1/2(u122)
  Saturation2/1 -> [uh121], bypass/2(u122)
  "op cold - bypass "/1 -> valvula 3/1(In1)
  "op hot - bypass "/1 -> valvula 1/1(In1)
  valvula 3/1(Out1) -> Saturation1/1
  valvula 1/1(Out1) -> Saturation2/1

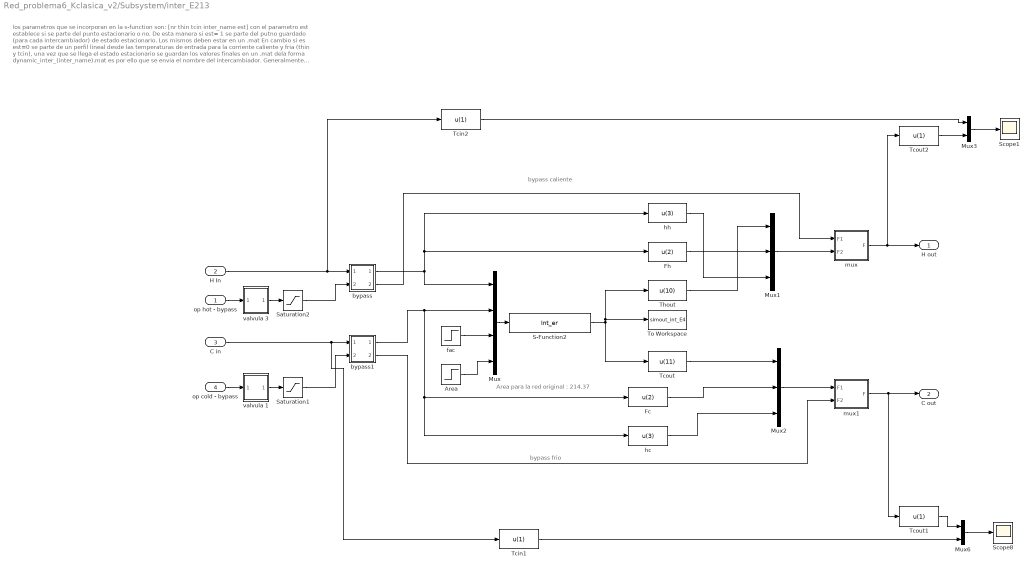
== system Red_problema6_Kclasica_v2/Subsystem/inter_E213 ==
  note: Area para la red original : 214.37
  note: bypass caliente
  note: bypass frio
  note: los parametros que se incorporan en la s-function son: [nr thin tcin inter_name est]
      | con el parametro est establece si se parte del punto estacionario o no. De esta manera si est= 1 se parte del putno guardado (para cada intercambiador) de estado estacionario. Los mismos deben estar en un .mat
      | En cambio si es est=0 se parte de un perfil lineal  desde las temperaturas de entrada para la corriente caliente y fria (thin y tcin), una vez que se llega el estado estacionario se guardan los valores finales en un .mat
      | dela forma dynamic_inter_(inter_name).mat   es por ello que se envia el nombre del intercambiador.
      | Generalmente para la primera vez que se corre la red se una est=0 para que llegue al estado estacionario y una vez que se alcanzó se vuelve a correr con est= 1 para hacer análisis de control
  "op hot - bypass " : Inport
  H In : Inport  Port=2
  C in : Inport  Port=3
  "op cold - bypass " : Inport  Port=4
  Area : Step  Time=8  Before=aE213  After=aE213  SampleTime=0
  Fc : Fcn  Expr=u(2)
  Fh : Fcn  Expr=u(2)
  Mux : Mux
  Mux1 : Mux  Inputs=3
  Mux2 : Mux  Inputs=3
  Mux3 : Mux  Inputs=2
  Mux6 : Mux  Inputs=2
  S-Function2 : S-Function  FunctionName=Int_er  Parameters=10 343 323 213 est  SFunctionDeploymentMode=off  EnableBusSupport=off
  Saturation1 : Saturate  UpperLimit=1  LowerLimit=0
  Saturation2 : Saturate  UpperLimit=1  LowerLimit=0
  Scope1 : Scope
  Scope8 : Scope
  Tcin1 : Fcn  Expr=u(1)
  Tcin2 : Fcn  Expr=u(1)
  Tcout : Fcn  Expr=u(11)
  Tcout1 : Fcn  Expr=u(1)
  Tcout2 : Fcn  Expr=u(1)
  Thout : Fcn  Expr=u(10)
  To Workspace : ToWorkspace  VariableName=simout_int_E4  SampleTime=-1
  bypass : Subsystem
  bypass1 : Subsystem
  fac : Step  After=0  SampleTime=0
  hc : Fcn  Expr=u(3)
  hh : Fcn  Expr=u(3)
  mux : Subsystem
  mux1 : Subsystem
  valvula 1 : Subsystem
  valvula 3 : Subsystem
  H out : Outport  VectorParamsAs1DForOutWhenUnconnected=off
  C out : Outport  Port=2  VectorParamsAs1DForOutWhenUnconnected=off
  wires:
  Tcin2/1 -> Mux3/1
  Tcout2/1 -> Mux3/2
  Mux3/1 -> Scope1/1
  Tcin1/1 -> Mux6/2
  Tcout1/1 -> Mux6/1
  Mux6/1 -> Scope8/1
  bypass1/2(" 2") -> mux1/2(F2)
  bypass1/1(" 1") -> Mux/2, Fc/1, hc/1
  mux1/1("F ") -> C out/1, Tcout1/1
  Mux2/1 -> mux1/1(F1)
  mux/1("F ") -> H out/1, Tcout2/1
  C in/1 -> bypass1/1(1), Tcin1/1
  bypass/2(" 2") -> mux/1(F1)
  Mux1/1 -> mux/2(F2)
  bypass/1(" 1") -> hh/1, Fh/1, Mux/1
  H In/1 -> bypass/1(1), Tcin2/1
  Area/1 -> Mux/4
  hh/1 -> Mux1/3
  hc/1 -> Mux2/3
  fac/1 -> Mux/3
  Mux/1 -> S-Function2/1
  S-Function2/1 -> Tcout/1, To Workspace/1, Thout/1
  Fh/1 -> Mux1/2
  Fc/1 -> Mux2/2
  Thout/1 -> Mux1/1
  Tcout/1 -> Mux2/1
  Saturation1/1 -> bypass1/2(u122)
  Saturation2/1 -> bypass/2(u122)
  "op hot - bypass "/1 -> valvula 3/1(In1)
  "op cold - bypass "/1 -> valvula 1/1(In1)
  valvula 1/1(Out1) -> Saturation1/1
  valvula 3/1(Out1) -> Saturation2/1

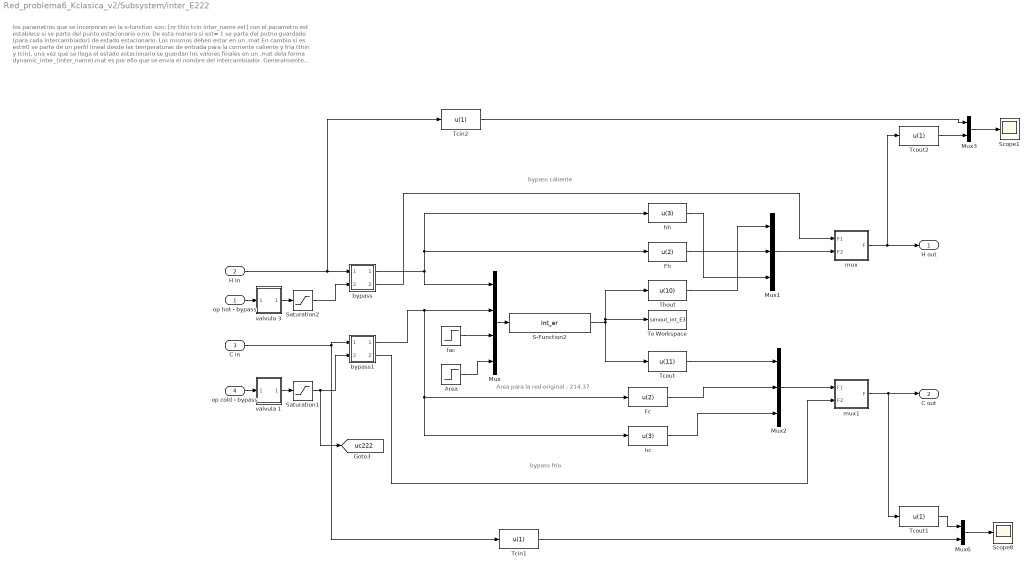
== system Red_problema6_Kclasica_v2/Subsystem/inter_E222 ==
  note: Area para la red original : 214.37
  note: bypass caliente
  note: bypass frio
  note: los parametros que se incorporan en la s-function son: [nr thin tcin inter_name est]
      | con el parametro est establece si se parte del punto estacionario o no. De esta manera si est= 1 se parte del putno guardado (para cada intercambiador) de estado estacionario. Los mismos deben estar en un .mat
      | En cambio si es est=0 se parte de un perfil lineal  desde las temperaturas de entrada para la corriente caliente y fria (thin y tcin), una vez que se llega el estado estacionario se guardan los valores finales en un .mat
      | dela forma dynamic_inter_(inter_name).mat   es por ello que se envia el nombre del intercambiador.
      | Generalmente para la primera vez que se corre la red se una est=0 para que llegue al estado estacionario y una vez que se alcanzó se vuelve a correr con est= 1 para hacer análisis de control
  "op hot - bypass " : Inport
  H In : Inport  Port=2
  C in : Inport  Port=3
  "op cold - bypass " : Inport  Port=4
  Area : Step  Time=8  Before=aE222  After=aE222  SampleTime=0
  Fc : Fcn  Expr=u(2)
  Fh : Fcn  Expr=u(2)
  Mux : Mux
  Mux1 : Mux  Inputs=3
  Mux2 : Mux  Inputs=3
  Mux3 : Mux  Inputs=2
  Mux6 : Mux  Inputs=2
  S-Function2 : S-Function  FunctionName=Int_er  Parameters=10 493 433 222 est  SFunctionDeploymentMode=off  EnableBusSupport=off
  Saturation1 : Saturate  UpperLimit=1  LowerLimit=0
  Saturation2 : Saturate  UpperLimit=1  LowerLimit=0
  Scope1 : Scope
  Scope8 : Scope
  Tcin1 : Fcn  Expr=u(1)
  Tcin2 : Fcn  Expr=u(1)
  Tcout : Fcn  Expr=u(11)
  Tcout1 : Fcn  Expr=u(1)
  Tcout2 : Fcn  Expr=u(1)
  Thout : Fcn  Expr=u(10)
  To Workspace : ToWorkspace  VariableName=simout_int_E3  SampleTime=-1
  bypass : Subsystem
  bypass1 : Subsystem
  fac : Step  After=0  SampleTime=0
  hc : Fcn  Expr=u(3)
  hh : Fcn  Expr=u(3)
  mux : Subsystem
  mux1 : Subsystem
  valvula 1 : Subsystem
  valvula 3 : Subsystem
  H out : Outport  VectorParamsAs1DForOutWhenUnconnected=off
  C out : Outport  Port=2  VectorParamsAs1DForOutWhenUnconnected=off
  tag scope: uc222=global
  wires:
  Tcin2/1 -> Mux3/1
  Tcout2/1 -> Mux3/2
  Mux3/1 -> Scope1/1
  Tcin1/1 -> Mux6/2
  Tcout1/1 -> Mux6/1
  Mux6/1 -> Scope8/1
  bypass1/2(" 2") -> mux1/2(F2)
  bypass1/1(" 1") -> Mux/2, Fc/1, hc/1
  mux1/1("F ") -> C out/1, Tcout1/1
  Mux2/1 -> mux1/1(F1)
  mux/1("F ") -> H out/1, Tcout2/1
  C in/1 -> bypass1/1(1), Tcin1/1
  bypass/2(" 2") -> mux/1(F1)
  Mux1/1 -> mux/2(F2)
  bypass/1(" 1") -> hh/1, Fh/1, Mux/1
  H In/1 -> bypass/1(1), Tcin2/1
  Area/1 -> Mux/4
  hh/1 -> Mux1/3
  hc/1 -> Mux2/3
  fac/1 -> Mux/3
  Mux/1 -> S-Function2/1
  S-Function2/1 -> To Workspace/1, Thout/1, Tcout/1
  Fh/1 -> Mux1/2
  Fc/1 -> Mux2/2
  Thout/1 -> Mux1/1
  Tcout/1 -> Mux2/1
  Saturation1/1 -> [uc222], bypass1/2(u122)
  Saturation2/1 -> bypass/2(u122)
  "op hot - bypass "/1 -> valvula 3/1(In1)
  "op cold - bypass "/1 -> valvula 1/1(In1)
  valvula 1/1(Out1) -> Saturation1/1
  valvula 3/1(Out1) -> Saturation2/1

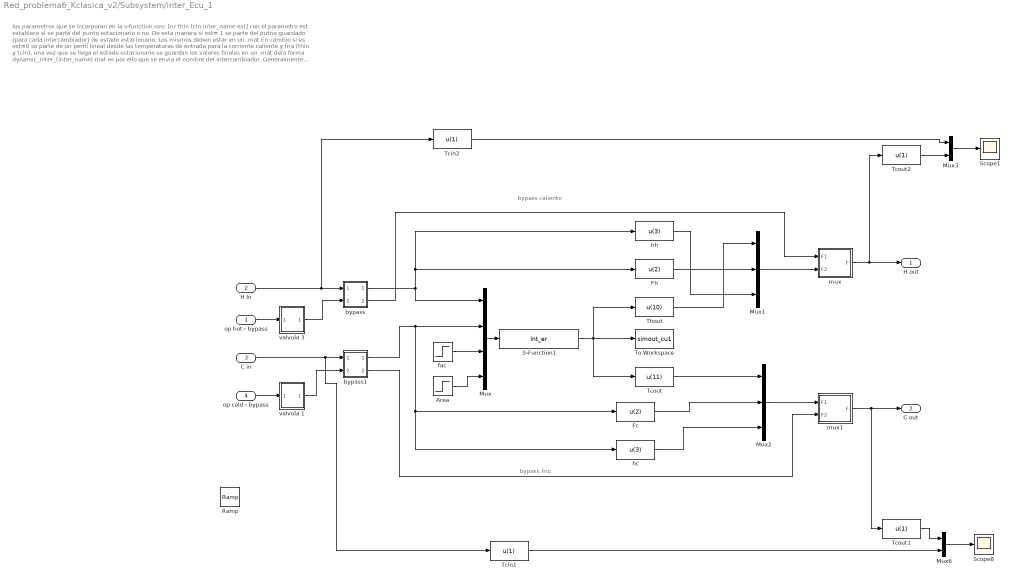
== system Red_problema6_Kclasica_v2/Subsystem/inter_Ecu_1 ==
  note: bypass caliente
  note: bypass frio
  note: los parametros que se incorporan en la s-function son: [nr thin tcin inter_name est]
      | con el parametro est establece si se parte del punto estacionario o no. De esta manera si est= 1 se parte del putno guardado (para cada intercambiador) de estado estacionario. Los mismos deben estar en un .mat
      | En cambio si es est=0 se parte de un perfil lineal  desde las temperaturas de entrada para la corriente caliente y fria (thin y tcin), una vez que se llega el estado estacionario se guardan los valores finales en un .mat
      | dela forma dynamic_inter_(inter_name).mat   es por ello que se envia el nombre del intercambiador.
      | Generalmente para la primera vez que se corre la red se una est=0 para que llegue al estado estacionario y una vez que se alcanzó se vuelve a correr con est= 1 para hacer análisis de control
  "op hot - bypass " : Inport
  H In : Inport  Port=2
  C in : Inport  Port=3
  "op cold - bypass " : Inport  Port=4
  Area : Step  Time=8  Before=aEcu1  After=aEcu1  SampleTime=0
  Fc : Fcn  Expr=u(2)
  Fh : Fcn  Expr=u(2)
  Mux : Mux
  Mux1 : Mux  Inputs=3
  Mux2 : Mux  Inputs=3
  Mux3 : Mux  Inputs=2
  Mux6 : Mux  Inputs=2
  Ramp : simulink/Sources/Ramp  slope=1  start=0  InitialOutput=0
  S-Function1 : S-Function  FunctionName=Int_er  Parameters=10 443 288 01 est  SFunctionDeploymentMode=off  EnableBusSupport=off
  Scope1 : Scope
  Scope8 : Scope
  Tcin1 : Fcn  Expr=u(1)
  Tcin2 : Fcn  Expr=u(1)
  Tcout : Fcn  Expr=u(11)
  Tcout1 : Fcn  Expr=u(1)
  Tcout2 : Fcn  Expr=u(1)
  Thout : Fcn  Expr=u(10)
  To Workspace : ToWorkspace  VariableName=simout_cu1  SampleTime=-1
  bypass : Subsystem
  bypass1 : Subsystem
  fac : Step  After=0  SampleTime=0
  hc : Fcn  Expr=u(3)
  hh : Fcn  Expr=u(3)
  mux : Subsystem
  mux1 : Subsystem
  valvula 1 : Subsystem
  valvula 3 : Subsystem
  H out : Outport  VectorParamsAs1DForOutWhenUnconnected=off
  C out : Outport  Port=2  VectorParamsAs1DForOutWhenUnconnected=off
  wires:
  Tcin2/1 -> Mux3/1
  Tcout2/1 -> Mux3/2
  Mux3/1 -> Scope1/1
  Tcin1/1 -> Mux6/2
  Tcout1/1 -> Mux6/1
  Mux6/1 -> Scope8/1
  bypass1/2(" 2") -> mux1/2(F2)
  bypass1/1(" 1") -> Mux/2, Fc/1, hc/1
  mux1/1("F ") -> C out/1, Tcout1/1
  Mux2/1 -> mux1/1(F1)
  C in/1 -> bypass1/1(1), Tcin1/1
  bypass/2(" 2") -> mux/1(F1)
  Mux1/1 -> mux/2(F2)
  bypass/1(" 1") -> hh/1, Fh/1, Mux/1
  H In/1 -> bypass/1(1), Tcin2/1
  Area/1 -> Mux/4
  hh/1 -> Mux1/3
  hc/1 -> Mux2/3
  fac/1 -> Mux/3
  Mux/1 -> S-Function1/1
  S-Function1/1 -> Thout/1, To Workspace/1, Tcout/1
  Fh/1 -> Mux1/2
  Fc/1 -> Mux2/2
  Thout/1 -> Mux1/1
  Tcout/1 -> Mux2/1
  "op hot - bypass "/1 -> valvula 3/1(In1)
  "op cold - bypass "/1 -> valvula 1/1(In1)
  mux/1("F ") -> H out/1, Tcout2/1
  valvula 1/1(Out1) -> bypass1/2(u122)
  valvula 3/1(Out1) -> bypass/2(u122)

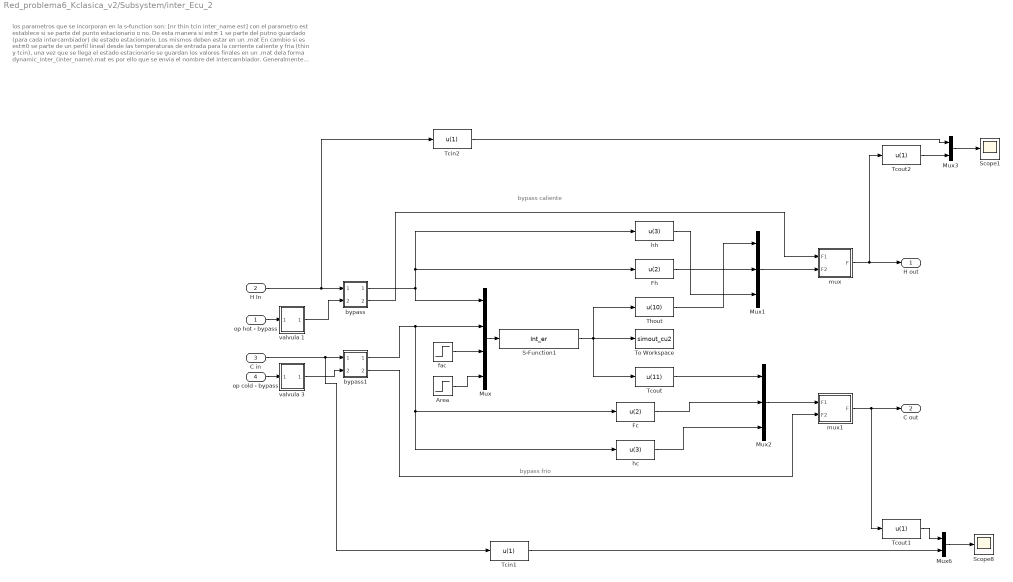
== system Red_problema6_Kclasica_v2/Subsystem/inter_Ecu_2 ==
  note: bypass caliente
  note: bypass frio
  note: los parametros que se incorporan en la s-function son: [nr thin tcin inter_name est]
      | con el parametro est establece si se parte del punto estacionario o no. De esta manera si est= 1 se parte del putno guardado (para cada intercambiador) de estado estacionario. Los mismos deben estar en un .mat
      | En cambio si es est=0 se parte de un perfil lineal  desde las temperaturas de entrada para la corriente caliente y fria (thin y tcin), una vez que se llega el estado estacionario se guardan los valores finales en un .mat
      | dela forma dynamic_inter_(inter_name).mat   es por ello que se envia el nombre del intercambiador.
      | Generalmente para la primera vez que se corre la red se una est=0 para que llegue al estado estacionario y una vez que se alcanzó se vuelve a correr con est= 1 para hacer análisis de control
  "op hot - bypass " : Inport
  H In : Inport  Port=2
  C in : Inport  Port=3
  "op cold - bypass " : Inport  Port=4
  Area : Step  Time=0  Before=aEcu2  After=aEcu2  SampleTime=0
  Fc : Fcn  Expr=u(2)
  Fh : Fcn  Expr=u(2)
  Mux : Mux
  Mux1 : Mux  Inputs=3
  Mux2 : Mux  Inputs=3
  Mux3 : Mux  Inputs=2
  Mux6 : Mux  Inputs=2
  S-Function1 : S-Function  FunctionName=Int_er  Parameters=10 343 288 02 est  SFunctionDeploymentMode=off  EnableBusSupport=off
  Scope1 : Scope
  Scope8 : Scope
  Tcin1 : Fcn  Expr=u(1)
  Tcin2 : Fcn  Expr=u(1)
  Tcout : Fcn  Expr=u(11)
  Tcout1 : Fcn  Expr=u(1)
  Tcout2 : Fcn  Expr=u(1)
  Thout : Fcn  Expr=u(10)
  To Workspace : ToWorkspace  VariableName=simout_cu2  SampleTime=-1
  bypass : Subsystem
  bypass1 : Subsystem
  fac : Step  After=0  SampleTime=0
  hc : Fcn  Expr=u(3)
  hh : Fcn  Expr=u(3)
  mux : Subsystem
  mux1 : Subsystem
  valvula 1 : Subsystem
  valvula 3 : Subsystem
  H out : Outport  VectorParamsAs1DForOutWhenUnconnected=off
  C out : Outport  Port=2  VectorParamsAs1DForOutWhenUnconnected=off
  wires:
  Tcin2/1 -> Mux3/1
  Tcout2/1 -> Mux3/2
  Mux3/1 -> Scope1/1
  Tcin1/1 -> Mux6/2
  Tcout1/1 -> Mux6/1
  Mux6/1 -> Scope8/1
  bypass1/2(" 2") -> mux1/2(F2)
  bypass1/1(" 1") -> Mux/2, Fc/1, hc/1
  mux1/1("F ") -> C out/1, Tcout1/1
  Mux2/1 -> mux1/1(F1)
  mux/1("F ") -> H out/1, Tcout2/1
  C in/1 -> bypass1/1(1), Tcin1/1
  bypass/2(" 2") -> mux/1(F1)
  Mux1/1 -> mux/2(F2)
  bypass/1(" 1") -> hh/1, Fh/1, Mux/1
  H In/1 -> bypass/1(1), Tcin2/1
  Area/1 -> Mux/4
  hh/1 -> Mux1/3
  hc/1 -> Mux2/3
  fac/1 -> Mux/3
  Mux/1 -> S-Function1/1
  S-Function1/1 -> Thout/1, To Workspace/1, Tcout/1
  Fh/1 -> Mux1/2
  Fc/1 -> Mux2/2
  Thout/1 -> Mux1/1
  Tcout/1 -> Mux2/1
  "op cold - bypass "/1 -> valvula 3/1(In1)
  "op hot - bypass "/1 -> valvula 1/1(In1)
  valvula 3/1(Out1) -> bypass1/2(u122)
  valvula 1/1(Out1) -> bypass/2(u122)

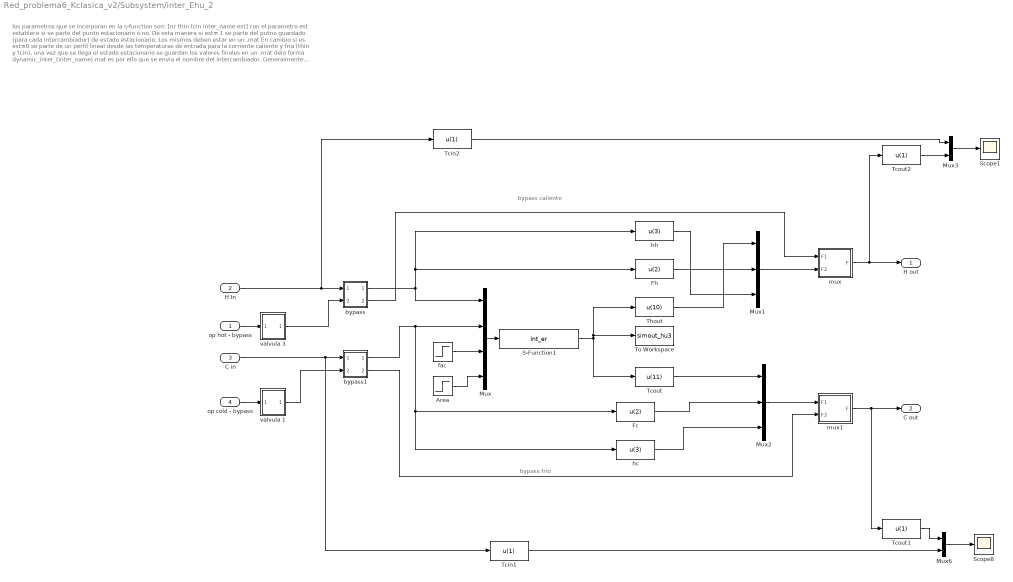
== system Red_problema6_Kclasica_v2/Subsystem/inter_Ehu_2 ==
  note: bypass caliente
  note: bypass frio
  note: los parametros que se incorporan en la s-function son: [nr thin tcin inter_name est]
      | con el parametro est establece si se parte del punto estacionario o no. De esta manera si est= 1 se parte del putno guardado (para cada intercambiador) de estado estacionario. Los mismos deben estar en un .mat
      | En cambio si es est=0 se parte de un perfil lineal  desde las temperaturas de entrada para la corriente caliente y fria (thin y tcin), una vez que se llega el estado estacionario se guardan los valores finales en un .mat
      | dela forma dynamic_inter_(inter_name).mat   es por ello que se envia el nombre del intercambiador.
      | Generalmente para la primera vez que se corre la red se una est=0 para que llegue al estado estacionario y una vez que se alcanzó se vuelve a correr con est= 1 para hacer análisis de control
  "op hot - bypass " : Inport
  H In : Inport  Port=2
  C in : Inport  Port=3
  "op cold - bypass " : Inport  Port=4
  Area : Step  Time=8  Before=aEhu2  After=aEhu2  SampleTime=0
  Fc : Fcn  Expr=u(2)
  Fh : Fcn  Expr=u(2)
  Mux : Mux
  Mux1 : Mux  Inputs=3
  Mux2 : Mux  Inputs=3
  Mux3 : Mux  Inputs=2
  Mux6 : Mux  Inputs=2
  S-Function1 : S-Function  FunctionName=Int_er  Parameters=10 523 471 03 est  SFunctionDeploymentMode=off  EnableBusSupport=off
  Scope1 : Scope
  Scope8 : Scope
  Tcin1 : Fcn  Expr=u(1)
  Tcin2 : Fcn  Expr=u(1)
  Tcout : Fcn  Expr=u(11)
  Tcout1 : Fcn  Expr=u(1)
  Tcout2 : Fcn  Expr=u(1)
  Thout : Fcn  Expr=u(10)
  To Workspace : ToWorkspace  VariableName=simout_hu3  SampleTime=-1
  bypass : Subsystem
  bypass1 : Subsystem
  fac : Step  After=0  SampleTime=0
  hc : Fcn  Expr=u(3)
  hh : Fcn  Expr=u(3)
  mux : Subsystem
  mux1 : Subsystem
  valvula 1 : Subsystem
  valvula 3 : Subsystem
  H out : Outport  VectorParamsAs1DForOutWhenUnconnected=off
  C out : Outport  Port=2  VectorParamsAs1DForOutWhenUnconnected=off
  wires:
  Tcin2/1 -> Mux3/1
  Tcout2/1 -> Mux3/2
  Mux3/1 -> Scope1/1
  Tcin1/1 -> Mux6/2
  Tcout1/1 -> Mux6/1
  Mux6/1 -> Scope8/1
  bypass1/2(" 2") -> mux1/2(F2)
  bypass1/1(" 1") -> Mux/2, Fc/1, hc/1
  mux1/1("F ") -> C out/1, Tcout1/1
  Mux2/1 -> mux1/1(F1)
  mux/1("F ") -> H out/1, Tcout2/1
  C in/1 -> bypass1/1(1), Tcin1/1
  bypass/2(" 2") -> mux/1(F1)
  Mux1/1 -> mux/2(F2)
  bypass/1(" 1") -> hh/1, Fh/1, Mux/1
  H In/1 -> bypass/1(1), Tcin2/1
  Area/1 -> Mux/4
  hh/1 -> Mux1/3
  hc/1 -> Mux2/3
  fac/1 -> Mux/3
  Mux/1 -> S-Function1/1
  S-Function1/1 -> Tcout/1, To Workspace/1, Thout/1
  Fh/1 -> Mux1/2
  Fc/1 -> Mux2/2
  Thout/1 -> Mux1/1
  Tcout/1 -> Mux2/1
  "op hot - bypass "/1 -> valvula 3/1(In1)
  "op cold - bypass "/1 -> valvula 1/1(In1)
  valvula 1/1(Out1) -> bypass1/2(u122)
  valvula 3/1(Out1) -> bypass/2(u122)

== system Red_problema6_Kclasica_v2/Subsystem/Corriente Hu1/valvula 3 ==
  In1 : Inport
  Gain : Gain  Gain=s1
  Gain1 : Gain  Gain=s1
  Integrator : Integrator  InitialCondition=[Tcuin fcu1 hcu]
  Sum : Sum  Inputs=|+-
  Out1 : Outport  VectorParamsAs1DForOutWhenUnconnected=off
  wires:
  Gain1/1 -> Sum/2
  Integrator/1 -> Out1/1, Gain1/1
  Sum/1 -> Integrator/1
  Gain/1 -> Sum/1
  In1/1 -> Gain/1

== system Red_problema6_Kclasica_v2/Subsystem/Corriente Hu2/valvula 3 ==
  In1 : Inport
  Gain : Gain  Gain=s1
  Gain1 : Gain  Gain=s1
  Integrator : Integrator  InitialCondition=[Tcuin fcu2 hcu]
  Sum : Sum  Inputs=|+-
  Out1 : Outport  VectorParamsAs1DForOutWhenUnconnected=off
  wires:
  Gain1/1 -> Sum/2
  Integrator/1 -> Out1/1, Gain1/1
  Sum/1 -> Integrator/1
  Gain/1 -> Sum/1
  In1/1 -> Gain/1

== system Red_problema6_Kclasica_v2/Subsystem/Corriente Hu3/valvula 3 ==
  In1 : Inport
  Gain : Gain  Gain=s1
  Gain1 : Gain  Gain=s1
  Integrator : Integrator  InitialCondition=[Thuin fhu2 hhu]
  Sum : Sum  Inputs=|+-
  Out1 : Outport  VectorParamsAs1DForOutWhenUnconnected=off
  wires:
  Gain1/1 -> Sum/2
  Integrator/1 -> Out1/1, Gain1/1
  Sum/1 -> Integrator/1
  Gain/1 -> Sum/1
  In1/1 -> Gain/1

== system Red_problema6_Kclasica_v2/Subsystem/inter_E112/bypass ==
  note: la corriente 1 es la que se introduce al intercambiador
  note: la corriete 2 es la corriente del byapass
  1 : Inport
  u122 : Inport  Port=2
  Add : Sum  Inputs=+-
  Mux : Mux  Inputs=3
  Mux1 : Mux  Inputs=3
  Product : Product
  T : Fcn  Expr=u(1)
  f : Fcn  Expr=u(2)
  h : Fcn  Expr=u(3)
  " 1" : Outport  VectorParamsAs1DForOutWhenUnconnected=off
  " 2" : Outport  Port=2  VectorParamsAs1DForOutWhenUnconnected=off
  wires:
  Mux1/1 -> " 2"/1
  Mux/1 -> " 1"/1
  T/1 -> Mux/1, Mux1/1
  h/1 -> Mux/3, Mux1/3
  Add/1 -> Mux/2
  1/1 -> f/1, h/1, T/1
  Product/1 -> Add/2, Mux1/2
  f/1 -> Product/2, Add/1
  u122/1 -> Product/1

== system Red_problema6_Kclasica_v2/Subsystem/inter_E112/bypass1 ==
  note: la corriete 2 es la corriente del byapass
  note: la corriente 1 es la que se introduce al intercambiador
  1 : Inport
  u122 : Inport  Port=2
  Add : Sum  Inputs=+-
  Mux : Mux  Inputs=3
  Mux1 : Mux  Inputs=3
  Product : Product
  T : Fcn  Expr=u(1)
  f : Fcn  Expr=u(2)
  h : Fcn  Expr=u(3)
  " 1" : Outport  VectorParamsAs1DForOutWhenUnconnected=off
  " 2" : Outport  Port=2  VectorParamsAs1DForOutWhenUnconnected=off
  wires:
  u122/1 -> Product/1
  f/1 -> Add/1, Product/2
  Product/1 -> Mux1/2, Add/2
  1/1 -> T/1, h/1, f/1
  Add/1 -> Mux/2
  h/1 -> Mux1/3, Mux/3
  T/1 -> Mux1/1, Mux/1
  Mux/1 -> " 1"/1
  Mux1/1 -> " 2"/1

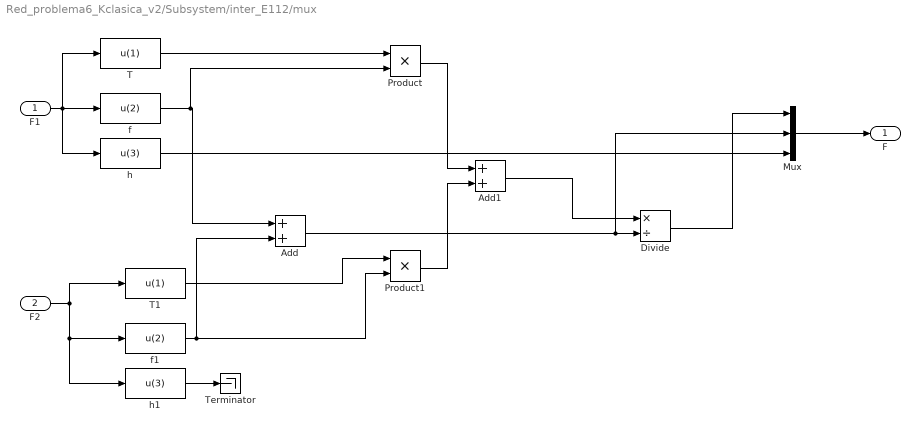
== system Red_problema6_Kclasica_v2/Subsystem/inter_E112/mux ==
  F1 : Inport
  F2 : Inport  Port=2
  Add : Sum
  Add1 : Sum
  Divide : Product  Inputs=*/
  Mux : Mux  Inputs=3
  Product : Product
  Product1 : Product
  T : Fcn  Expr=u(1)
  T1 : Fcn  Expr=u(1)
  Terminator : Terminator
  f : Fcn  Expr=u(2)
  f1 : Fcn  Expr=u(2)
  h : Fcn  Expr=u(3)
  h1 : Fcn  Expr=u(3)
  "F " : Outport  VectorParamsAs1DForOutWhenUnconnected=off
  wires:
  Mux/1 -> "F "/1
  F1/1 -> f/1, h/1, T/1
  f/1 -> Product/2, Add/1
  F2/1 -> h1/1, f1/1, T1/1
  T/1 -> Product/1
  Product/1 -> Add1/1
  T1/1 -> Product1/1
  f1/1 -> Add/2, Product1/2
  Product1/1 -> Add1/2
  Add1/1 -> Divide/1
  Add/1 -> Mux/2, Divide/2
  Divide/1 -> Mux/1
  h/1 -> Mux/3
  h1/1 -> Terminator/1

== system Red_problema6_Kclasica_v2/Subsystem/inter_E112/mux1 ==
  F1 : Inport
  F2 : Inport  Port=2
  Add : Sum
  Add1 : Sum
  Divide : Product  Inputs=*/
  Mux : Mux  Inputs=3
  Product : Product
  Product1 : Product
  T : Fcn  Expr=u(1)
  T1 : Fcn  Expr=u(1)
  Terminator : Terminator
  f : Fcn  Expr=u(2)
  f1 : Fcn  Expr=u(2)
  h : Fcn  Expr=u(3)
  h1 : Fcn  Expr=u(3)
  "F " : Outport  VectorParamsAs1DForOutWhenUnconnected=off
  wires:
  h/1 -> Mux/3
  Divide/1 -> Mux/1
  Add/1 -> Divide/2, Mux/2
  Add1/1 -> Divide/1
  Product1/1 -> Add1/2
  f1/1 -> Product1/2, Add/2
  T1/1 -> Product1/1
  Product/1 -> Add1/1
  T/1 -> Product/1
  F2/1 -> T1/1, f1/1, h1/1
  f/1 -> Add/1, Product/2
  F1/1 -> T/1, h/1, f/1
  Mux/1 -> "F "/1
  h1/1 -> Terminator/1

== system Red_problema6_Kclasica_v2/Subsystem/inter_E112/valvula 1 ==
  In1 : Inport
  Gain : Gain  Gain=s1
  Gain1 : Gain  Gain=s1
  Integrator : Integrator
  Sum : Sum  Inputs=|+-
  Out1 : Outport  VectorParamsAs1DForOutWhenUnconnected=off
  wires:
  Gain1/1 -> Sum/2
  Integrator/1 -> Out1/1, Gain1/1
  Sum/1 -> Integrator/1
  Gain/1 -> Sum/1
  In1/1 -> Gain/1
